simulink model "LastModel"  (R2016a)
settings: Solver=VariableStepAuto  StartTime=0.0  StopTime=0.0001  FixedStep=0.001  RelTol=1e-3
libraries: elec_lib x14, fl_lib x6, nesl_utility x6
settings Model: Creator=syf  LastModifiedBy=syf
settings DebuggingCC: AlgebraicLoopMsg=none  ArtificialAlgebraicLoopMsg=none

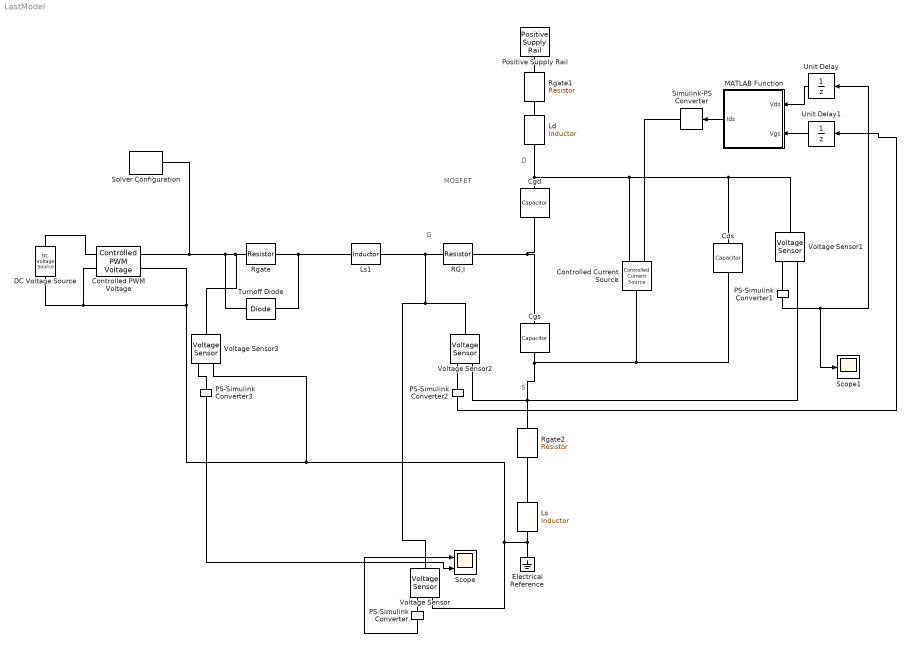
== system LastModel ==
  note: MOSFET
  note: S
  note: D
  note: G
  Cds : elec_lib/Passive Devices/Capacitor  enable_table=0  c=100 pF  Cvec=[ 1e-5 1e-6 ] F  Vvec=[ 0 10 ] V  CV_table_symmetry=1  C_tol=5  enable_C_tol=0  tol_distribution=1  nSigma=4  r=0 Ohm  g=0 1/Ohm  initV=0 V  enable_operating_limits=0  operating_limit_action=2  max_working_voltage_range=[ -25 25 ] V  power_rating=1 W  enable_faults=0  fault_action=1  Cscale_faulted=100  R_faulted=0.001 Ohm  G_faulted=0 1/Ohm  tau_fault=0.001 s  enable_temporal_fault=0  t_fault=1 s  enable_behavioral_fault=0  max_permissible_voltage_range=[ -100 100 ] V  t_fail_on_voltage=1 s
  Cgd : elec_lib/Passive Devices/Capacitor  enable_table=0  c=10 pF  Cvec=[ 1e-5 1e-6 ] F  Vvec=[ 0 10 ] V  CV_table_symmetry=1  C_tol=5  enable_C_tol=0  tol_distribution=1  nSigma=4  r=0 Ohm  g=0 1/Ohm  initV=0 V  enable_operating_limits=0  operating_limit_action=2  max_working_voltage_range=[ -25 25 ] V  power_rating=1 W  enable_faults=0  fault_action=1  Cscale_faulted=100  R_faulted=0.001 Ohm  G_faulted=0 1/Ohm  tau_fault=0.001 s  enable_temporal_fault=0  t_fault=1 s  enable_behavioral_fault=0  max_permissible_voltage_range=[ -100 100 ] V  t_fail_on_voltage=1 s
  Cgs : elec_lib/Passive Devices/Capacitor  enable_table=0  c=190 pF  Cvec=[ 1e-5 1e-6 ] F  Vvec=[ 0 10 ] V  CV_table_symmetry=1  C_tol=5  enable_C_tol=0  tol_distribution=1  nSigma=4  r=0 Ohm  g=0 1/Ohm  initV=0 V  enable_operating_limits=0  operating_limit_action=2  max_working_voltage_range=[ -25 25 ] V  power_rating=1 W  enable_faults=0  fault_action=1  Cscale_faulted=100  R_faulted=0.001 Ohm  G_faulted=0 1/Ohm  tau_fault=0.001 s  enable_temporal_fault=0  t_fault=1 s  enable_behavioral_fault=0  max_permissible_voltage_range=[ -100 100 ] V  t_fail_on_voltage=1 s
  Controlled Current Source : fl_lib/Electrical/Electrical Sources/Controlled Current Source
  Controlled PWM Voltage : elec_lib/Actuators & Drivers/Drivers/Controlled PWM Voltage  F=50 kHz  TD=0 s  pulse_width_offset=0 s  Vmin=0 V  Vmax=6 V  Vm=6 V  pwm_or_av=1  event_type=1  sample_time=1e-6 s
  DC Voltage Source : elec_lib/Additional Components/SPICE-Compatible Components/Sources/DC Voltage Source  DC=3 V
  Electrical Reference : fl_lib/Electrical/Electrical Elements/Electrical Reference
  Ld : elec_lib/Passive Devices/Inductor  l=10 nH  L_tol=20  enable_L_tol=0  tol_distribution=1  nSigma=4  r=0 Ohm  g=0 1/Ohm  initI=0 A  enable_operating_limits=0  operating_limit_action=2  max_working_current=1 A  power_rating=1 W  enable_faults=0  fault_action=1  lambdaPercent=50  k_faulted=0.9999 Ohm  turnsShort=0  openCct=0  groundShort=0  groundShortG=0 1/Ohm  tau_fault=0.001 s  enable_temporal_fault=0  t_fault=1 s  enable_behavioral_fault=0  max_permissible_voltage=100 V  n_fail_on_voltage=1  max_permissible_current=1 A  t_fail_on_current=1 s
  Ls : elec_lib/Passive Devices/Inductor  l=2 nH  L_tol=20  enable_L_tol=0  tol_distribution=1  nSigma=4  r=0 Ohm  g=0 1/Ohm  initI=0 A  enable_operating_limits=0  operating_limit_action=2  max_working_current=1 A  power_rating=1 W  enable_faults=0  fault_action=1  lambdaPercent=50  k_faulted=0.9999 Ohm  turnsShort=0  openCct=0  groundShort=0  groundShortG=0 1/Ohm  tau_fault=0.001 s  enable_temporal_fault=0  t_fault=1 s  enable_behavioral_fault=0  max_permissible_voltage=100 V  n_fail_on_voltage=1  max_permissible_current=1 A  t_fail_on_current=1 s
  Ls1 : elec_lib/Passive Devices/Inductor  l=5 nH  L_tol=20  enable_L_tol=0  tol_distribution=1  nSigma=4  r=0 Ohm  g=0 1/Ohm  initI=0 A  enable_operating_limits=0  operating_limit_action=2  max_working_current=1 A  power_rating=1 W  enable_faults=0  fault_action=1  lambdaPercent=50  k_faulted=0.9999 Ohm  turnsShort=0  openCct=0  groundShort=0  groundShortG=0 1/Ohm  tau_fault=0.001 s  enable_temporal_fault=0  t_fault=1 s  enable_behavioral_fault=0  max_permissible_voltage=100 V  n_fail_on_voltage=1  max_permissible_current=1 A  t_fail_on_current=1 s
  MATLAB Function : MATLAB Function  TreatAsAtomicUnit=on
  PS-Simulink Converter{,1..3} (4 alike) : nesl_utility/PS-Simulink Converter  PhysicalDomain=network_engine_domain  SubClassName=ps_output  LeftPortType=input  RightPortType=output  PseudoPeriodic=off  Frequencies=[]  Unit=1  AffineConversion=off
  Positive Supply Rail : elec_lib/Sources/Positive Supply Rail  v0=300 V
  RG,I : elec_lib/Passive Devices/Resistor  R=1.5 Ohm  R_tol=5  enable_R_tol=0  tol_distribution=1  nSigma=4  enable_operating_limits=0  operating_limit_action=2  max_working_voltage=100 V  power_rating=1 W  enable_faults=0  fault_action=1  R_faulted=Inf Ohm  enable_temporal_fault=0  t_fault=1 s  enable_behavioral_fault=0  max_permissible_current=1 A  t_fail_on_current=1 s  noise_mode=0  sample_time=0.001 s  repeatability=1  auto_seed=3674442472  user_seed=0  Tdevice=25 degC  alpha=0.00393 1/K  Tmeas=25 degC  thermal_mass=100 J/K  initial_temperature=25 degC  power_derating_T1=70 degC  power_derating_T2=155 degC  operating_temperature_range_vec=[ -50 150 ] degC
  Rgate : elec_lib/Passive Devices/Resistor  R=7 Ohm  R_tol=5  enable_R_tol=0  tol_distribution=1  nSigma=4  enable_operating_limits=0  operating_limit_action=2  max_working_voltage=100 V  power_rating=1 W  enable_faults=0  fault_action=1  R_faulted=Inf Ohm  enable_temporal_fault=0  t_fault=1 s  enable_behavioral_fault=0  max_permissible_current=1 A  t_fail_on_current=1 s  noise_mode=0  sample_time=0.001 s  repeatability=1  auto_seed=2586302551  user_seed=0  Tdevice=25 degC  alpha=0.00393 1/K  Tmeas=25 degC  thermal_mass=100 J/K  initial_temperature=25 degC  power_derating_T1=70 degC  power_derating_T2=155 degC  operating_temperature_range_vec=[ -50 150 ] degC
  Rgate1 : elec_lib/Passive Devices/Resistor  R=10 Ohm  R_tol=5  enable_R_tol=0  tol_distribution=1  nSigma=4  enable_operating_limits=0  operating_limit_action=2  max_working_voltage=100 V  power_rating=1 W  enable_faults=0  fault_action=1  R_faulted=Inf Ohm  enable_temporal_fault=0  t_fault=1 s  enable_behavioral_fault=0  max_permissible_current=1 A  t_fail_on_current=1 s  noise_mode=0  sample_time=0.001 s  repeatability=1  auto_seed=1401209772  user_seed=0  Tdevice=25 degC  alpha=0.00393 1/K  Tmeas=25 degC  thermal_mass=100 J/K  initial_temperature=25 degC  power_derating_T1=70 degC  power_derating_T2=155 degC  operating_temperature_range_vec=[ -50 150 ] degC
  Rgate2 : elec_lib/Passive Devices/Resistor  R=10 Ohm  R_tol=5  enable_R_tol=0  tol_distribution=1  nSigma=4  enable_operating_limits=0  operating_limit_action=2  max_working_voltage=100 V  power_rating=1 W  enable_faults=0  fault_action=1  R_faulted=Inf Ohm  enable_temporal_fault=0  t_fault=1 s  enable_behavioral_fault=0  max_permissible_current=1 A  t_fail_on_current=1 s  noise_mode=0  sample_time=0.001 s  repeatability=1  auto_seed=1671570447  user_seed=0  Tdevice=25 degC  alpha=0.00393 1/K  Tmeas=25 degC  thermal_mass=100 J/K  initial_temperature=25 degC  power_derating_T1=70 degC  power_derating_T2=155 degC  operating_temperature_range_vec=[ -50 150 ] degC
  Scope : Scope  NumInputPorts=2
  Scope1 : Scope
  Simulink-PS Converter : nesl_utility/Simulink-PS Converter  PhysicalDomain=network_engine_domain  SubClassName=ps_input  LeftPortType=input  RightPortType=output  PseudoPeriodic=off  Frequencies=[]  NoiseDistribution=none  NoiseParameters=[]  Unit=1  AffineConversion=off  InputFiltering=off  SimscapeFilterOrder=1  InputFilterTimeConstant=0.001  UdotUserProvided=1
  Solver Configuration : nesl_utility/Solver Configuration  PhysicalDomain=network_engine_domain  SubClassName=solver  LeftPortType=input  RightPortType=generic  Accelerate=off  Tones=[]  Harmonics=[]  SimulateNoise=off  Profile=off  UseLocalSampling=off  EnableSwitchedLinearOptims=on  FrequencyDomain=off  UseCCode=off  RelTol=0.001  AbsTol=1e-06  MinStep=1e-09  ToWorkspace=off  RevertToSquareIcSolve=off  NumHomotopyIterations=100  PhasorMode=off  PhasorModeNumHarmonics=1  OverrideAbsTol=off  DoDC=off  ResidualTolerance=1e-09  UseLocalSolver=off  LocalSolverChoice=NE_BACKWARD_EULER_ADVANCER  LocalSolverSampleTime=0.001  DoFixedCost=off  MaxNonlinIter=3  MaxModeIter=2  LinearAlgebra=Sparse  DelaysMemoryBudget=1024  AutomaticFiltering=on  FilteringTimeConstant=0.001
  Turnoff Diode : elec_lib/Semiconductor Devices/Diode  ModelType=1  Vf=0.6 V  Ron=0.3 Ohm  Goff=1e-8 S  Rz=0.3 Ohm  Vz=50 V  C_PWL=5 pF  prmExp=1  I12=[ 0.0137 0.545 ] A  V12=[ 0.6 0.7 ] V  I1=0.0137 A  V1=0.6 V  RS=0.01 Ohm  IS=1e-12 A  Tmeas=25 degC  ec=1  BV=Inf V  C_param=1  CJ0=5 pF  VJ=1 V  Mgrad=0.5  Vvec=[ 0.1 10 100 ] V  Cvec=[ 3.5 1 0.4 ] pF  FC=0.5  Q_param=1  Irrm=-7.15 A  iF=4 A  didt=-750 A/us  trr=115 ns  TT=50 ns  tau=100 ns  T_param=1  IS_T2=1.25e-7 A  I1_T2=0.245 A  V1_T2=0.5 V  Tmeas2=125 degC  EG_param=1  EG=1.11 eV  XTI_param=1  XTI=3  dBVdT=0 V/K  Tdevice=25 degC  Rth=[ 0 10 ] K/W  thermal_mass_parameterization=1  thermal_mass=[ 0 1 ] J/K  thermal_time_constant=[ 0 10 ] s  thermal_mass_initial_temperatures=[ 25 25 ] degC
  Unit Delay : UnitDelay  SampleTime=0.0001
  Unit Delay1 : UnitDelay  SampleTime=0.0001
  Voltage Sensor{,1..3} (4 alike) : fl_lib/Electrical/Electrical Sensors/Voltage Sensor
  wires:
  PS-Simulink Converter/1 -> Scope/1
  MATLAB Function/1(Ids) -> Simulink-PS Converter/1
  Unit Delay/1 -> MATLAB Function/1(Vds)
  Unit Delay1/1 -> MATLAB Function/2(Vgs)
  PS-Simulink Converter1/1 -> Scope1/1, Unit Delay/1
  PS-Simulink Converter2/1 -> Unit Delay1/1
  PS-Simulink Converter3/1 -> Scope/2
  connections:
  Cds/LConn1 -- Ld/RConn1 -- Cgd/LConn1 -- Controlled Current Source/RConn2 -- Voltage Sensor1/LConn1
  Voltage Sensor2/RConn2 -- Voltage Sensor1/RConn2 -- Rgate2/LConn1 -- Cgs/RConn1 -- Controlled Current Source/LConn1 -- Cds/RConn1
  Cgd/RConn1 -- RG,I/RConn1 -- Cgs/LConn1
  Ld/LConn1 -- Rgate1/RConn1
  Electrical Reference/LConn1 -- Ls/RConn1 -- Controlled PWM Voltage/RConn2 -- DC Voltage Source/RConn1 -- Controlled PWM Voltage/LConn2 -- Voltage Sensor3/RConn2 -- Voltage Sensor/RConn2
  Rgate/RConn1 -- Turnoff Diode/LConn1 -- Ls1/LConn1
  Rgate/LConn1 -- Controlled PWM Voltage/RConn1 -- Solver Configuration/RConn1 -- Turnoff Diode/RConn1 -- Voltage Sensor3/LConn1
  Voltage Sensor/RConn1 -- PS-Simulink Converter/LConn1
  Simulink-PS Converter/RConn1 -- Controlled Current Source/RConn1
  PS-Simulink Converter1/LConn1 -- Voltage Sensor1/RConn1
  PS-Simulink Converter2/LConn1 -- Voltage Sensor2/RConn1
  Voltage Sensor3/RConn1 -- PS-Simulink Converter3/LConn1
  Rgate1/LConn1 -- Positive Supply Rail/RConn1
  DC Voltage Source/LConn1 -- Controlled PWM Voltage/LConn1
  Voltage Sensor/LConn1 -- Ls1/RConn1 -- RG,I/LConn1 -- Voltage Sensor2/LConn1
  Rgate2/RConn1 -- Ls/LConn1

== matlab function LastModel/MATLAB Function ==
  data: Vds input; Ids output; Vgs input
function Ids = fcn(Vds, Vgs)
b1=2.035;
c1=0.124;
d1=1.159;
e1=-0.204;
b2=2.054;
c2=0.153;
m1=30.972;
n1=-4.48;
l1=4.316e-3;
l2=-1.091e-3;
h1=3.771e-3;
h2=-7.872e-3;
T=125;
k1=0.283;
k2=7.114;
Vgd=Vgs-Vds;

K1_T=k1*(1-l1*(T-25));
K2_T=k2*(1-l2*(T-25));
P1_T=(1-h1*(T-25));
P2_T=(1-h2*(T-25));


if Vds>0
    Ids=  K1_T*log(1+exp((Vgs-b1)/c1))*(((m1+n1*Vgs)*Vds)/(1+P1_T*(d1+e1*Vgs)*Vds));
else
    Ids= K2_T*log(1+exp((Vgd-b2)/c2))*(Vds/(1-P2_T*Vds));
end
